simulink model "testbench_rearwheel_parking"  (R2015a)
settings: Solver=ode3  StartTime=0.0  StopTime=inf  RelTol=1e-3
undefined symbols (not defined in the file or in its folder): sigbuilder_block
libraries: legoev3lib x6
settings Model: SimulationMode=external  ExtModeTrigDuration=2  Creator=Shobhit  LastModifiedBy=Keshav
settings OptimizationCC: OptimizeModelRefInitCode=on  LifeSpan=1
settings DebuggingCC: UnderspecifiedInitializationDetection=Classic  MergeDetectMultiDrivingBlocksExec=none
settings HardwareCC: ProdLargestAtomicInteger=Long  ProdLargestAtomicFloat=Float  ProdEndianess=LittleEndian  ProdHWDeviceType=ARM Compatible->ARM 9
settings RTWCC: SystemTargetFile=realtime.tlc  GenerateMakefile=off  TemplateMakefile=realtime.tmf  Description=Run on Target Hardware  RTWVerbose=off
settings ERTTargetCC: CombineOutputUpdateFcns=off  ERTSrcFileBannerTemplate=realtime_code_template.cgt  ERTHdrFileBannerTemplate=realtime_code_template.cgt  ERTDataSrcFileTemplate=realtime_code_template.cgt  ERTDataHdrFileTemplate=realtime_code_template.cgt  ERTCustomFileTemplate=realtime_file_process.tlc

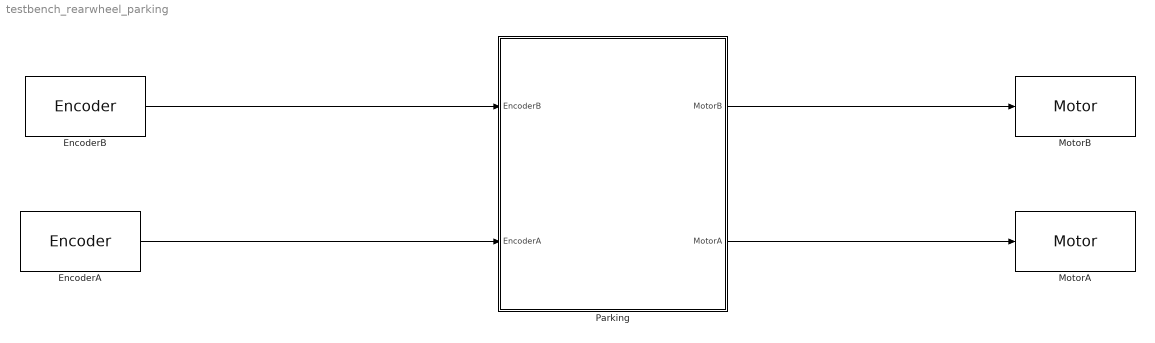
== system testbench_rearwheel_parking ==
  EncoderA : legoev3lib/Encoder  portNumber=A  opMode=No reset  sampleTime=0.1
  EncoderB : legoev3lib/Encoder  portNumber=B  opMode=No reset  sampleTime=0.1
  MotorA : legoev3lib/Motor  sportNumber=A  sstopAction=Brake
  MotorB : legoev3lib/Motor  sportNumber=B  sstopAction=Brake
  Parking : Subsystem
  wires:
  EncoderB/1 -> Parking/1(EncoderB)
  EncoderA/1 -> Parking/2(EncoderA)
  Parking/1(MotorB) -> MotorB/1
  Parking/2(MotorA) -> MotorA/1

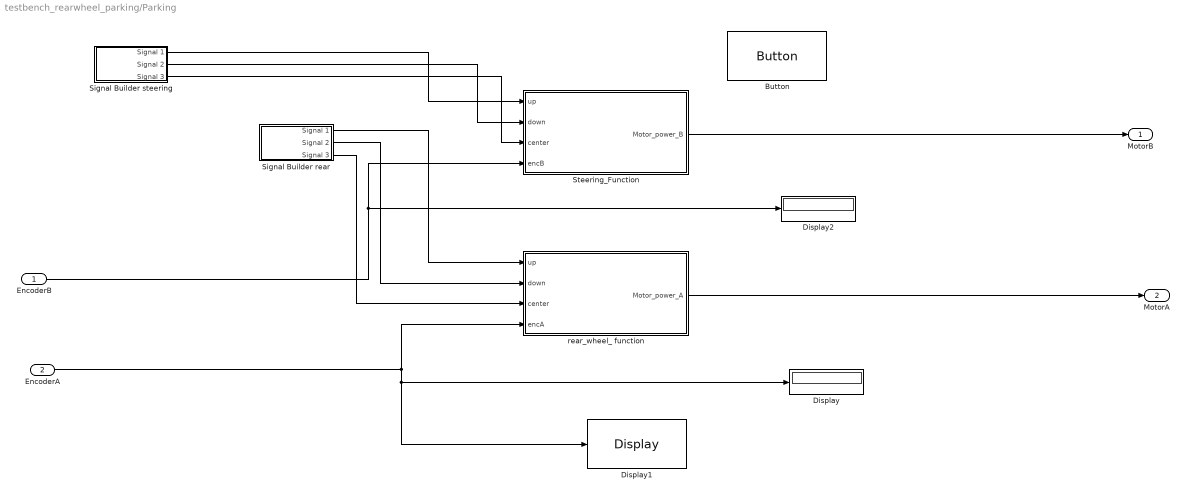
== system testbench_rearwheel_parking/Parking ==
  EncoderB : Inport
  EncoderA : Inport  Port=2
  " Steering_Function" : MATLAB Function  TreatAsAtomicUnit=on
  Button : legoev3lib/Button  buttonType=Up  sampleTime=0.1
  Display : Display
      settings: Format=decimal (Stored Integer)
  Display1 : legoev3lib/Display  slcdStr=enc A  slcdLine=1  slcdFormat=Decimal
  Display2 : Display
      settings: Format=decimal (Stored Integer)
  Signal Builder rear : Subsystem  Tag=STV Subsys  LoadFcn=sigbuilder_block('load');  StartFcn=sigbuilder_block('start');  StopFcn=sigbuilder_block('stop');  ClipboardFcn=sigbuilder_block('clipboard');  mask(Sigbuilder block){}
      mask help: Simulink:masks:SigbuilderBlock_MD
      mask init:
      | if ~strcmp(get_param(bdroot(gcbh),'SimulationStatus'),'stopped') tuvar = sigbuilder_block('maskInit'); end
      settings: CopyFcn=sigbuilder_block('copy');  DeleteFcn=sigbuilder_block('delete');  ModelCloseFcn=sigbuilder_block('modelClose');  PreSaveFcn=sigbuilder_block('preSave');  PauseFcn=sigbuilder_block('pause');  ContinueFcn=sigbuilder_block('continue');  NameChangeFcn=sigbuilder_block('namechange');  OpenFcn=sigbuilder_block('open',[438 199 636 400 ]);  CloseFcn=sigbuilder_block('close');
      mask Display: plot(0, 0, 100, 100,[2, 2, 32, 32, 2], [68, 8, 8, 68, 68],[32, 2], [38, 38], [32, 19, 2],[53, 60, 44], [32, 17, 17, 2],[16, 16, 31, 31]);txt = getActiveGroup(gcbh);text(2, 100, txt,'verticalAlignment', 'top');
  Signal Builder steering : Subsystem  Tag=STV Subsys  LoadFcn=sigbuilder_block('load');  StartFcn=sigbuilder_block('start');  StopFcn=sigbuilder_block('stop');  ClipboardFcn=sigbuilder_block('clipboard');  mask(Sigbuilder block){}
      mask help: Simulink:masks:SigbuilderBlock_MD
      mask init:
      | if ~strcmp(get_param(bdroot(gcbh),'SimulationStatus'),'stopped') tuvar = sigbuilder_block('maskInit'); end
      settings: CopyFcn=sigbuilder_block('copy');  DeleteFcn=sigbuilder_block('delete');  ModelCloseFcn=sigbuilder_block('modelClose');  PreSaveFcn=sigbuilder_block('preSave');  PauseFcn=sigbuilder_block('pause');  ContinueFcn=sigbuilder_block('continue');  NameChangeFcn=sigbuilder_block('namechange');  OpenFcn=sigbuilder_block('open',[438 199 636 400 ]);  CloseFcn=sigbuilder_block('close');
      mask Display: plot(0, 0, 100, 100,[2, 2, 32, 32, 2], [68, 8, 8, 68, 68],[32, 2], [38, 38], [32, 19, 2],[53, 60, 44], [32, 17, 17, 2],[16, 16, 31, 31]);txt = getActiveGroup(gcbh);text(2, 100, txt,'verticalAlignment', 'top');
  rear_wheel_ function : MATLAB Function  TreatAsAtomicUnit=on
  MotorB : Outport
  MotorA : Outport  Port=2
  wires:
  " Steering_Function"/1(Motor_power_B) -> MotorB/1
  Signal Builder steering/3(Signal 3) -> " Steering_Function"/3(center)
  rear_wheel_ function/1(Motor_power_A) -> MotorA/1
  Signal Builder rear/3(Signal 3) -> rear_wheel_ function/3(center)
  Signal Builder steering/1(Signal 1) -> " Steering_Function"/1(up)
  Signal Builder rear/2(Signal 2) -> rear_wheel_ function/2(down)
  EncoderA/1 -> Display1/1, Display/1, rear_wheel_ function/4(encA)
  Signal Builder steering/2(Signal 2) -> " Steering_Function"/2(down)
  Signal Builder rear/1(Signal 1) -> rear_wheel_ function/1(up)
  EncoderB/1 -> " Steering_Function"/4(encB), Display2/1

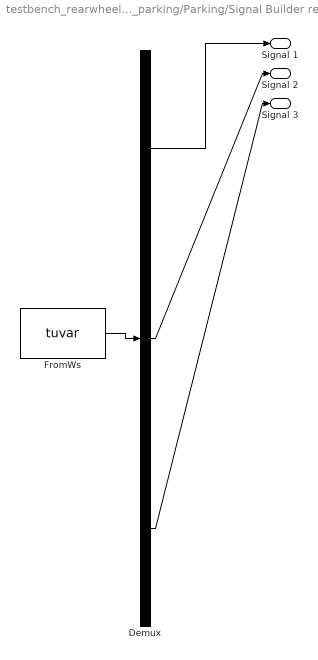
== system testbench_rearwheel_parking/Parking/Signal Builder rear ==
  Demux : Demux  Tag=STV Demux  Outputs=3
  FromWs : FromWorkspace  Tag=STV FromWs  VariableName=tuvar  SampleTime=0
      SigBuilderData=|
      | common.afterFinalStr = 'Extrapolate'
      | common.sampleTime = 0
      | dataSet.timeRange = [0 25]
      | dataSet.name = 'Move'
      | sbobj.Groups.Name = 'Move'
      | sbobj.Groups.Signals(1).Name = 'Signal 1'
      | sbobj.Groups.Signals(1).XData = [0 2.5 2.5 6.75 6.75 25]
      | sbobj.Groups.Signals(1).YData = [0 0 1 1 0 0]
      | sbobj.Groups.Signals(2).Name = 'Signal 2'
      | sbobj.Groups.Signals(2).XData = [0 9 9 13 13 25]
      | sbobj.Groups.Signals(2).YData = [0 0 1 1 0 0]
      | sbobj.Groups.Signals(3).Name = 'Signal 3'
      | sbobj.Groups.Signals(3).XData = [0 16.8 16.8 22.85 22.85 25]
      | sbobj.Groups.Signals(3).YData = [0 0 1 1 0 0]
      | sbobj.Groups.TimeRange = [0 25]
  Signal 1 : Outport  Tag=STV Outport
  Signal 2 : Outport  Tag=STV Outport  Port=2
  Signal 3 : Outport  Tag=STV Outport  Port=3
  wires:
  Demux/1 -> Signal 1/1
  FromWs/1 -> Demux/1
  Demux/2 -> Signal 2/1
  Demux/3 -> Signal 3/1

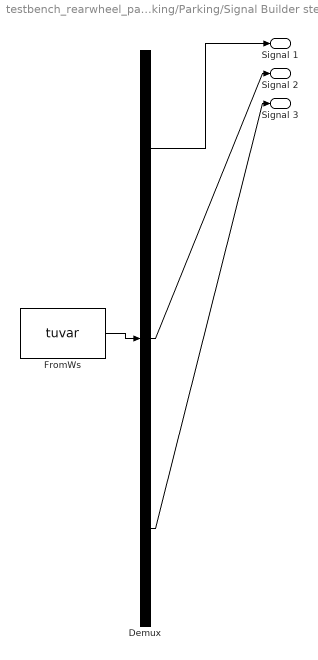
== system testbench_rearwheel_parking/Parking/Signal Builder steering ==
  Demux : Demux  Tag=STV Demux  Outputs=3
  FromWs : FromWorkspace  Tag=STV FromWs  VariableName=tuvar  SampleTime=0
      SigBuilderData=|
      | common.afterFinalStr = 'Extrapolate'
      | common.sampleTime = 0
      | dataSet.timeRange = [0 20]
      | dataSet.name = 'Steering'
      | sbobj.Groups.Name = 'Steering'
      | sbobj.Groups.Signals(1).Name = 'Signal 1'
      | sbobj.Groups.Signals(1).XData = [0 0.12 0.12 2.5 2.5 20]
      | sbobj.Groups.Signals(1).YData = [0 0 1 1 0 0]
      | sbobj.Groups.Signals(2).Name = 'Signal 2'
      | sbobj.Groups.Signals(2).XData = [0 6.75 6.75 9 9 20]
      | sbobj.Groups.Signals(2).YData = [0 0 1 1 0 0]
      | sbobj.Groups.Signals(3).Name = 'Signal 3'
      | sbobj.Groups.Signals(3).XData = [0 13.1 13.1 15.9 15.9 20]
      | sbobj.Groups.Signals(3).YData = [0 0 1 1 0 0]
      | sbobj.Groups.TimeRange = [0 20]
  Signal 1 : Outport  Tag=STV Outport
  Signal 2 : Outport  Tag=STV Outport  Port=2
  Signal 3 : Outport  Tag=STV Outport  Port=3
  wires:
  Demux/2 -> Signal 2/1
  FromWs/1 -> Demux/1
  Demux/1 -> Signal 1/1
  Demux/3 -> Signal 3/1

== matlab function testbench_rearwheel_parking/Parking/ Steering_Function ==
  data: up input; down input; center input; Motor_power_B output; encB input
function Motor_power_B=fcn(up,down,center,encB)
%#codegen
if(up==1)&&(encB>=-400)
   Motor_power_B=-70;
elseif(down==1)&&(encB<=400)
   Motor_power_B=70;
elseif (center==1)&&(encB>=5)
 %%  while(encB~=0)
   Motor_power_B=-70;
else
   Motor_power_B=0;
end
end

== matlab function testbench_rearwheel_parking/Parking/rear_wheel_ function ==
  data: Motor_power_A output; up input; down input; center input; encA input
function Motor_power_A=fcn(up, down,center,encA)
%#codegen
if (up==1)&&(encA>=-240)
  Motor_power_A = -30;
elseif (down==1)&&(encA>=-500)
     Motor_power_A = -30;
elseif (center==1)&&(encA<=-445)
    Motor_power_A=30;
else
    Motor_power_A=0; 
end
end
